simulink model "IEEE34_SPSload"  (R2021b)
settings: Solver=ode4  StartTime=0.0  StopTime=5  FixedStep=50e-6  RelTol=1e-3
PreLoadFcn:
  | pGain = 0.05; % Gain of random perturbation (pu)
  | pGainAP = 0.01; % Gain of sinusoidal active power variation (pu)
  | pGainRP = 0.01; % Gain of sinusoidal reactive power variation (pu)
  | pFreqAP = 0.03; % Frequency of sinusoidal active power variation (Hz)
  | pFreqRP = 0.03; % Frequency of sinusoidal reactive power variation (Hz)
  | 
  | init_IEEE34nodetestfeeder;
InitFcn:
  | pGain = 0.05; % Gain of random perturbation (pu)
  | pGainAP = 0.01; % Gain of sinusoidal active power variation (pu)
  | pGainRP = 0.01; % Gain of sinusoidal reactive power variation (pu)
  | pFreqAP = 0.03; % Frequency of sinusoidal active power variation (Hz)
  | pFreqRP = 0.03; % Frequency of sinusoidal reactive power variation (Hz)
  | 
  | init_IEEE34nodetestfeeder;
values from neighbouring files (symbols this model uses):
  fNom = f    (= 60)    [init_IEEE34nodetestfeeder.m]
  loadcoeff = 1.0    (= 1)    [init_IEEE34nodetestfeeder.m]
  Ts = 50e-6    (= 5e-05)    [init_IEEE34nodetestfeeder.m]
  vNomMV = VsubL    (= 24900)    [init_IEEE34nodetestfeeder.m]
  VsubL = 24.9e3    (= 24900)    [init_IEEE34nodetestfeeder.m]
  VxfmL = 4.16e3    (= 4160)    [init_IEEE34nodetestfeeder.m]
undefined symbols (not defined in the file or in its folder): Ac, Bc, Cc, Dc, find_system, j
libraries: spsSeriesRLCBranchLib x418, spsGroundLib x242, simulink_extras x176, spsVoltageMeasurementLib x106, spsRMSLib x96, spsControlledCurrentSourceLib x94, spsThreePhaseVIMeasurementLib x37, spsMutualInductanceLib x24, spsCurrentMeasurementLib x12, spsOnDelayLib x12, spsLinearTransformerLib x6, spsControlledVoltageSourceLib x6
(part 30 of 33)

== system IEEE34_SPSload/SM_IEEE34/DL_820-822/Load B/model/Positive Sequence current/TF_P ==
  In1 : Inport
  State-Space : StateSpace  A=Ac  B=Bc  C=Cc  D=Dc  InitialCondition=x0c
  Out1 : Outport  VectorParamsAs1DForOutWhenUnconnected=off
  wires:
  State-Space/1 -> Out1/1
  In1/1 -> State-Space/1

== system IEEE34_SPSload/SM_IEEE34/DL_820-822/Load B/model/Positive Sequence current/TF_Q ==
  In1 : Inport
  State-Space : StateSpace  A=Ac  B=Bc  C=Cc  D=Dc  InitialCondition=x0c
  Out1 : Outport  VectorParamsAs1DForOutWhenUnconnected=off
  wires:
  In1/1 -> State-Space/1
  State-Space/1 -> Out1/1

== system IEEE34_SPSload/SM_IEEE34/DL_824-1/Load B/model/PLL/adaptive filter ==
  u : Inport
  freq (Hz) : Inport  Port=2
  Gain : Gain  Gain=2*pi*2*0.707*2
  Gain1 : Gain  Gain=2*pi*2
  Product1 : Product  Inputs=***  RndMeth=Zero
  Product2 : Product  Inputs=**  RndMeth=Zero
  Product3 : Product  Inputs=***  RndMeth=Zero
  Sum1 : Sum  Inputs=+--  InputSameDT=on  SaturateOnIntegerOverflow=on  OutDataTypeStr=Inherit: Same as first input
  integrator1 : Integrator
  integrator2 : Integrator
  y : Outport  VectorParamsAs1DForOutWhenUnconnected=off
  wires:
  Product1/1 -> Sum1/2
  u/1 -> Product3/3
  freq (Hz)/1 -> Gain/1, Gain1/1
  Gain1/1 -> Product1/3, Product1/2, Product3/2, Product3/1
  Product3/1 -> Sum1/1
  integrator1/1 -> Product1/1, y/1
  Gain/1 -> Product2/2
  Product2/1 -> Sum1/3
  Sum1/1 -> integrator2/1
  integrator2/1 -> Product2/1, integrator1/1

== system IEEE34_SPSload/SM_IEEE34/DL_824-1/Load B/model/PLL/adaptive mean ==
  u : Inport
  freq (Hz) : Inport  Port=2
  Fcn : Fcn  Expr=u(1)+1e-6
  Math Function : Math  Operator=reciprocal  SignedPower=on  SaturateOnIntegerOverflow=on
  Product1 : Product  Inputs=**  RndMeth=Zero
  Sum : Sum  Inputs=+-  InputSameDT=on  SaturateOnIntegerOverflow=on  OutDataTypeStr=Inherit: Same as first input
  Variable Transport Delay : VariableTransportDelay  MaximumDelay=1/40  MaximumPoints=4096
  integrator : Integrator
  y : Outport  VectorParamsAs1DForOutWhenUnconnected=off
  wires:
  Product1/1 -> y/1
  u/1 -> integrator/1
  Sum/1 -> Product1/1
  integrator/1 -> Variable Transport Delay/1, Sum/1
  Variable Transport Delay/1 -> Sum/2
  Math Function/1 -> Variable Transport Delay/2
  freq (Hz)/1 -> Fcn/1
  Fcn/1 -> Math Function/1, Product1/2

== system IEEE34_SPSload/SM_IEEE34/DL_824-1/Load B/model/Positive Sequence current/TF_P ==
  In1 : Inport
  State-Space : StateSpace  A=Ac  B=Bc  C=Cc  D=Dc  InitialCondition=x0c
  Out1 : Outport  VectorParamsAs1DForOutWhenUnconnected=off
  wires:
  State-Space/1 -> Out1/1
  In1/1 -> State-Space/1

== system IEEE34_SPSload/SM_IEEE34/DL_824-1/Load B/model/Positive Sequence current/TF_Q ==
  In1 : Inport
  State-Space : StateSpace  A=Ac  B=Bc  C=Cc  D=Dc  InitialCondition=x0c
  Out1 : Outport  VectorParamsAs1DForOutWhenUnconnected=off
  wires:
  In1/1 -> State-Space/1
  State-Space/1 -> Out1/1

== system IEEE34_SPSload/SM_IEEE34/DL_824-2/Load B/model/PLL/adaptive filter ==
  u : Inport
  freq (Hz) : Inport  Port=2
  Gain : Gain  Gain=2*pi*2*0.707*2
  Gain1 : Gain  Gain=2*pi*2
  Product1 : Product  Inputs=***  RndMeth=Zero
  Product2 : Product  Inputs=**  RndMeth=Zero
  Product3 : Product  Inputs=***  RndMeth=Zero
  Sum1 : Sum  Inputs=+--  InputSameDT=on  SaturateOnIntegerOverflow=on  OutDataTypeStr=Inherit: Same as first input
  integrator1 : Integrator
  integrator2 : Integrator
  y : Outport  VectorParamsAs1DForOutWhenUnconnected=off
  wires:
  integrator2/1 -> integrator1/1, Product2/1
  Sum1/1 -> integrator2/1
  Product2/1 -> Sum1/3
  Gain/1 -> Product2/2
  integrator1/1 -> y/1, Product1/1
  Product3/1 -> Sum1/1
  Gain1/1 -> Product3/1, Product3/2, Product1/2, Product1/3
  freq (Hz)/1 -> Gain1/1, Gain/1
  u/1 -> Product3/3
  Product1/1 -> Sum1/2

== system IEEE34_SPSload/SM_IEEE34/DL_824-2/Load B/model/PLL/adaptive mean ==
  u : Inport
  freq (Hz) : Inport  Port=2
  Fcn : Fcn  Expr=u(1)+1e-6
  Math Function : Math  Operator=reciprocal  SignedPower=on  SaturateOnIntegerOverflow=on
  Product1 : Product  Inputs=**  RndMeth=Zero
  Sum : Sum  Inputs=+-  InputSameDT=on  SaturateOnIntegerOverflow=on  OutDataTypeStr=Inherit: Same as first input
  Variable Transport Delay : VariableTransportDelay  MaximumDelay=1/40  MaximumPoints=4096
  integrator : Integrator
  y : Outport  VectorParamsAs1DForOutWhenUnconnected=off
  wires:
  Fcn/1 -> Product1/2, Math Function/1
  freq (Hz)/1 -> Fcn/1
  Math Function/1 -> Variable Transport Delay/2
  Variable Transport Delay/1 -> Sum/2
  integrator/1 -> Sum/1, Variable Transport Delay/1
  Sum/1 -> Product1/1
  u/1 -> integrator/1
  Product1/1 -> y/1

== system IEEE34_SPSload/SM_IEEE34/DL_824-2/Load B/model/Positive Sequence current/TF_P ==
  In1 : Inport
  State-Space : StateSpace  A=Ac  B=Bc  C=Cc  D=Dc  InitialCondition=x0c
  Out1 : Outport  VectorParamsAs1DForOutWhenUnconnected=off
  wires:
  In1/1 -> State-Space/1
  State-Space/1 -> Out1/1

== system IEEE34_SPSload/SM_IEEE34/DL_824-2/Load B/model/Positive Sequence current/TF_Q ==
  In1 : Inport
  State-Space : StateSpace  A=Ac  B=Bc  C=Cc  D=Dc  InitialCondition=x0c
  Out1 : Outport  VectorParamsAs1DForOutWhenUnconnected=off
  wires:
  State-Space/1 -> Out1/1
  In1/1 -> State-Space/1

== system IEEE34_SPSload/SM_IEEE34/DL_824-826/Load B/model/PLL/adaptive filter ==
  u : Inport
  freq (Hz) : Inport  Port=2
  Gain : Gain  Gain=2*pi*2*0.707*2
  Gain1 : Gain  Gain=2*pi*2
  Product1 : Product  Inputs=***  RndMeth=Zero
  Product2 : Product  Inputs=**  RndMeth=Zero
  Product3 : Product  Inputs=***  RndMeth=Zero
  Sum1 : Sum  Inputs=+--  InputSameDT=on  SaturateOnIntegerOverflow=on  OutDataTypeStr=Inherit: Same as first input
  integrator1 : Integrator
  integrator2 : Integrator
  y : Outport  VectorParamsAs1DForOutWhenUnconnected=off
  wires:
  Product1/1 -> Sum1/2
  u/1 -> Product3/3
  freq (Hz)/1 -> Gain/1, Gain1/1
  Gain1/1 -> Product1/3, Product1/2, Product3/2, Product3/1
  Product3/1 -> Sum1/1
  integrator1/1 -> Product1/1, y/1
  Gain/1 -> Product2/2
  Product2/1 -> Sum1/3
  Sum1/1 -> integrator2/1
  integrator2/1 -> Product2/1, integrator1/1

== system IEEE34_SPSload/SM_IEEE34/DL_824-826/Load B/model/PLL/adaptive mean ==
  u : Inport
  freq (Hz) : Inport  Port=2
  Fcn : Fcn  Expr=u(1)+1e-6
  Math Function : Math  Operator=reciprocal  SignedPower=on  SaturateOnIntegerOverflow=on
  Product1 : Product  Inputs=**  RndMeth=Zero
  Sum : Sum  Inputs=+-  InputSameDT=on  SaturateOnIntegerOverflow=on  OutDataTypeStr=Inherit: Same as first input
  Variable Transport Delay : VariableTransportDelay  MaximumDelay=1/40  MaximumPoints=4096
  integrator : Integrator
  y : Outport  VectorParamsAs1DForOutWhenUnconnected=off
  wires:
  Product1/1 -> y/1
  u/1 -> integrator/1
  Sum/1 -> Product1/1
  integrator/1 -> Variable Transport Delay/1, Sum/1
  Variable Transport Delay/1 -> Sum/2
  Math Function/1 -> Variable Transport Delay/2
  freq (Hz)/1 -> Fcn/1
  Fcn/1 -> Math Function/1, Product1/2

== system IEEE34_SPSload/SM_IEEE34/DL_824-826/Load B/model/Positive Sequence current/TF_P ==
  In1 : Inport
  State-Space : StateSpace  A=Ac  B=Bc  C=Cc  D=Dc  InitialCondition=x0c
  Out1 : Outport  VectorParamsAs1DForOutWhenUnconnected=off
  wires:
  State-Space/1 -> Out1/1
  In1/1 -> State-Space/1

== system IEEE34_SPSload/SM_IEEE34/DL_824-826/Load B/model/Positive Sequence current/TF_Q ==
  In1 : Inport
  State-Space : StateSpace  A=Ac  B=Bc  C=Cc  D=Dc  InitialCondition=x0c
  Out1 : Outport  VectorParamsAs1DForOutWhenUnconnected=off
  wires:
  In1/1 -> State-Space/1
  State-Space/1 -> Out1/1

== system IEEE34_SPSload/SM_IEEE34/DL_824-828/Load B/model/PLL/adaptive filter ==
  u : Inport
  freq (Hz) : Inport  Port=2
  Gain : Gain  Gain=2*pi*2*0.707*2
  Gain1 : Gain  Gain=2*pi*2
  Product1 : Product  Inputs=***  RndMeth=Zero
  Product2 : Product  Inputs=**  RndMeth=Zero
  Product3 : Product  Inputs=***  RndMeth=Zero
  Sum1 : Sum  Inputs=+--  InputSameDT=on  SaturateOnIntegerOverflow=on  OutDataTypeStr=Inherit: Same as first input
  integrator1 : Integrator
  integrator2 : Integrator
  y : Outport  VectorParamsAs1DForOutWhenUnconnected=off
  wires:
  Product1/1 -> Sum1/2
  u/1 -> Product3/3
  freq (Hz)/1 -> Gain/1, Gain1/1
  Gain1/1 -> Product1/3, Product1/2, Product3/2, Product3/1
  Product3/1 -> Sum1/1
  integrator1/1 -> Product1/1, y/1
  Gain/1 -> Product2/2
  Product2/1 -> Sum1/3
  Sum1/1 -> integrator2/1
  integrator2/1 -> Product2/1, integrator1/1

== system IEEE34_SPSload/SM_IEEE34/DL_824-828/Load B/model/PLL/adaptive mean ==
  u : Inport
  freq (Hz) : Inport  Port=2
  Fcn : Fcn  Expr=u(1)+1e-6
  Math Function : Math  Operator=reciprocal  SignedPower=on  SaturateOnIntegerOverflow=on
  Product1 : Product  Inputs=**  RndMeth=Zero
  Sum : Sum  Inputs=+-  InputSameDT=on  SaturateOnIntegerOverflow=on  OutDataTypeStr=Inherit: Same as first input
  Variable Transport Delay : VariableTransportDelay  MaximumDelay=1/40  MaximumPoints=4096
  integrator : Integrator
  y : Outport  VectorParamsAs1DForOutWhenUnconnected=off
  wires:
  Product1/1 -> y/1
  u/1 -> integrator/1
  Sum/1 -> Product1/1
  integrator/1 -> Variable Transport Delay/1, Sum/1
  Variable Transport Delay/1 -> Sum/2
  Math Function/1 -> Variable Transport Delay/2
  freq (Hz)/1 -> Fcn/1
  Fcn/1 -> Math Function/1, Product1/2

== system IEEE34_SPSload/SM_IEEE34/DL_824-828/Load B/model/Positive Sequence current/TF_P ==
  In1 : Inport
  State-Space : StateSpace  A=Ac  B=Bc  C=Cc  D=Dc  InitialCondition=x0c
  Out1 : Outport  VectorParamsAs1DForOutWhenUnconnected=off
  wires:
  State-Space/1 -> Out1/1
  In1/1 -> State-Space/1

== system IEEE34_SPSload/SM_IEEE34/DL_824-828/Load B/model/Positive Sequence current/TF_Q ==
  In1 : Inport
  State-Space : StateSpace  A=Ac  B=Bc  C=Cc  D=Dc  InitialCondition=x0c
  Out1 : Outport  VectorParamsAs1DForOutWhenUnconnected=off
  wires:
  In1/1 -> State-Space/1
  State-Space/1 -> Out1/1

== system IEEE34_SPSload/SM_IEEE34/DL_828-1/Load B/model/PLL/adaptive filter ==
  u : Inport
  freq (Hz) : Inport  Port=2
  Gain : Gain  Gain=2*pi*2*0.707*2
  Gain1 : Gain  Gain=2*pi*2
  Product1 : Product  Inputs=***  RndMeth=Zero
  Product2 : Product  Inputs=**  RndMeth=Zero
  Product3 : Product  Inputs=***  RndMeth=Zero
  Sum1 : Sum  Inputs=+--  InputSameDT=on  SaturateOnIntegerOverflow=on  OutDataTypeStr=Inherit: Same as first input
  integrator1 : Integrator
  integrator2 : Integrator
  y : Outport  VectorParamsAs1DForOutWhenUnconnected=off
  wires:
  integrator2/1 -> integrator1/1, Product2/1
  Sum1/1 -> integrator2/1
  Product2/1 -> Sum1/3
  Gain/1 -> Product2/2
  integrator1/1 -> y/1, Product1/1
  Product3/1 -> Sum1/1
  Gain1/1 -> Product3/1, Product3/2, Product1/2, Product1/3
  freq (Hz)/1 -> Gain1/1, Gain/1
  u/1 -> Product3/3
  Product1/1 -> Sum1/2

== system IEEE34_SPSload/SM_IEEE34/DL_828-1/Load B/model/PLL/adaptive mean ==
  u : Inport
  freq (Hz) : Inport  Port=2
  Fcn : Fcn  Expr=u(1)+1e-6
  Math Function : Math  Operator=reciprocal  SignedPower=on  SaturateOnIntegerOverflow=on
  Product1 : Product  Inputs=**  RndMeth=Zero
  Sum : Sum  Inputs=+-  InputSameDT=on  SaturateOnIntegerOverflow=on  OutDataTypeStr=Inherit: Same as first input
  Variable Transport Delay : VariableTransportDelay  MaximumDelay=1/40  MaximumPoints=4096
  integrator : Integrator
  y : Outport  VectorParamsAs1DForOutWhenUnconnected=off
  wires:
  Fcn/1 -> Product1/2, Math Function/1
  freq (Hz)/1 -> Fcn/1
  Math Function/1 -> Variable Transport Delay/2
  Variable Transport Delay/1 -> Sum/2
  integrator/1 -> Sum/1, Variable Transport Delay/1
  Sum/1 -> Product1/1
  u/1 -> integrator/1
  Product1/1 -> y/1

== system IEEE34_SPSload/SM_IEEE34/DL_828-1/Load B/model/Positive Sequence current/TF_P ==
  In1 : Inport
  State-Space : StateSpace  A=Ac  B=Bc  C=Cc  D=Dc  InitialCondition=x0c
  Out1 : Outport  VectorParamsAs1DForOutWhenUnconnected=off
  wires:
  In1/1 -> State-Space/1
  State-Space/1 -> Out1/1

== system IEEE34_SPSload/SM_IEEE34/DL_828-1/Load B/model/Positive Sequence current/TF_Q ==
  In1 : Inport
  State-Space : StateSpace  A=Ac  B=Bc  C=Cc  D=Dc  InitialCondition=x0c
  Out1 : Outport  VectorParamsAs1DForOutWhenUnconnected=off
  wires:
  State-Space/1 -> Out1/1
  In1/1 -> State-Space/1

== system IEEE34_SPSload/SM_IEEE34/DL_828-830/Load B/model/PLL/adaptive filter ==
  u : Inport
  freq (Hz) : Inport  Port=2
  Gain : Gain  Gain=2*pi*2*0.707*2
  Gain1 : Gain  Gain=2*pi*2
  Product1 : Product  Inputs=***  RndMeth=Zero
  Product2 : Product  Inputs=**  RndMeth=Zero
  Product3 : Product  Inputs=***  RndMeth=Zero
  Sum1 : Sum  Inputs=+--  InputSameDT=on  SaturateOnIntegerOverflow=on  OutDataTypeStr=Inherit: Same as first input
  integrator1 : Integrator
  integrator2 : Integrator
  y : Outport  VectorParamsAs1DForOutWhenUnconnected=off
  wires:
  Product1/1 -> Sum1/2
  u/1 -> Product3/3
  freq (Hz)/1 -> Gain/1, Gain1/1
  Gain1/1 -> Product1/3, Product1/2, Product3/2, Product3/1
  Product3/1 -> Sum1/1
  integrator1/1 -> Product1/1, y/1
  Gain/1 -> Product2/2
  Product2/1 -> Sum1/3
  Sum1/1 -> integrator2/1
  integrator2/1 -> Product2/1, integrator1/1

== system IEEE34_SPSload/SM_IEEE34/DL_828-830/Load B/model/PLL/adaptive mean ==
  u : Inport
  freq (Hz) : Inport  Port=2
  Fcn : Fcn  Expr=u(1)+1e-6
  Math Function : Math  Operator=reciprocal  SignedPower=on  SaturateOnIntegerOverflow=on
  Product1 : Product  Inputs=**  RndMeth=Zero
  Sum : Sum  Inputs=+-  InputSameDT=on  SaturateOnIntegerOverflow=on  OutDataTypeStr=Inherit: Same as first input
  Variable Transport Delay : VariableTransportDelay  MaximumDelay=1/40  MaximumPoints=4096
  integrator : Integrator
  y : Outport  VectorParamsAs1DForOutWhenUnconnected=off
  wires:
  Product1/1 -> y/1
  u/1 -> integrator/1
  Sum/1 -> Product1/1
  integrator/1 -> Variable Transport Delay/1, Sum/1
  Variable Transport Delay/1 -> Sum/2
  Math Function/1 -> Variable Transport Delay/2
  freq (Hz)/1 -> Fcn/1
  Fcn/1 -> Math Function/1, Product1/2

== system IEEE34_SPSload/SM_IEEE34/DL_828-830/Load B/model/Positive Sequence current/TF_P ==
  In1 : Inport
  State-Space : StateSpace  A=Ac  B=Bc  C=Cc  D=Dc  InitialCondition=x0c
  Out1 : Outport  VectorParamsAs1DForOutWhenUnconnected=off
  wires:
  State-Space/1 -> Out1/1
  In1/1 -> State-Space/1

== system IEEE34_SPSload/SM_IEEE34/DL_828-830/Load B/model/Positive Sequence current/TF_Q ==
  In1 : Inport
  State-Space : StateSpace  A=Ac  B=Bc  C=Cc  D=Dc  InitialCondition=x0c
  Out1 : Outport  VectorParamsAs1DForOutWhenUnconnected=off
  wires:
  In1/1 -> State-Space/1
  State-Space/1 -> Out1/1

== system IEEE34_SPSload/SM_IEEE34/DL_832-1/Load A/model/PLL/adaptive filter ==
  u : Inport
  freq (Hz) : Inport  Port=2
  Gain : Gain  Gain=2*pi*2*0.707*2
  Gain1 : Gain  Gain=2*pi*2
  Product1 : Product  Inputs=***  RndMeth=Zero
  Product2 : Product  Inputs=**  RndMeth=Zero
  Product3 : Product  Inputs=***  RndMeth=Zero
  Sum1 : Sum  Inputs=+--  InputSameDT=on  SaturateOnIntegerOverflow=on  OutDataTypeStr=Inherit: Same as first input
  integrator1 : Integrator
  integrator2 : Integrator
  y : Outport  VectorParamsAs1DForOutWhenUnconnected=off
  wires:
  integrator2/1 -> integrator1/1, Product2/1
  Sum1/1 -> integrator2/1
  Product2/1 -> Sum1/3
  Gain/1 -> Product2/2
  integrator1/1 -> y/1, Product1/1
  Product3/1 -> Sum1/1
  Gain1/1 -> Product3/1, Product3/2, Product1/2, Product1/3
  freq (Hz)/1 -> Gain1/1, Gain/1
  u/1 -> Product3/3
  Product1/1 -> Sum1/2

== system IEEE34_SPSload/SM_IEEE34/DL_832-1/Load A/model/PLL/adaptive mean ==
  u : Inport
  freq (Hz) : Inport  Port=2
  Fcn : Fcn  Expr=u(1)+1e-6
  Math Function : Math  Operator=reciprocal  SignedPower=on  SaturateOnIntegerOverflow=on
  Product1 : Product  Inputs=**  RndMeth=Zero
  Sum : Sum  Inputs=+-  InputSameDT=on  SaturateOnIntegerOverflow=on  OutDataTypeStr=Inherit: Same as first input
  Variable Transport Delay : VariableTransportDelay  MaximumDelay=1/40  MaximumPoints=4096
  integrator : Integrator
  y : Outport  VectorParamsAs1DForOutWhenUnconnected=off
  wires:
  Fcn/1 -> Product1/2, Math Function/1
  freq (Hz)/1 -> Fcn/1
  Math Function/1 -> Variable Transport Delay/2
  Variable Transport Delay/1 -> Sum/2
  integrator/1 -> Sum/1, Variable Transport Delay/1
  Sum/1 -> Product1/1
  u/1 -> integrator/1
  Product1/1 -> y/1

== system IEEE34_SPSload/SM_IEEE34/DL_832-1/Load A/model/Positive Sequence current/TF_P ==
  In1 : Inport
  State-Space : StateSpace  A=Ac  B=Bc  C=Cc  D=Dc  InitialCondition=x0c
  Out1 : Outport  VectorParamsAs1DForOutWhenUnconnected=off
  wires:
  In1/1 -> State-Space/1
  State-Space/1 -> Out1/1

== system IEEE34_SPSload/SM_IEEE34/DL_832-1/Load A/model/Positive Sequence current/TF_Q ==
  In1 : Inport
  State-Space : StateSpace  A=Ac  B=Bc  C=Cc  D=Dc  InitialCondition=x0c
  Out1 : Outport  VectorParamsAs1DForOutWhenUnconnected=off
  wires:
  State-Space/1 -> Out1/1
  In1/1 -> State-Space/1

== system IEEE34_SPSload/SM_IEEE34/DL_832-1/Load B/model/PLL/adaptive filter ==
  u : Inport
  freq (Hz) : Inport  Port=2
  Gain : Gain  Gain=2*pi*2*0.707*2
  Gain1 : Gain  Gain=2*pi*2
  Product1 : Product  Inputs=***  RndMeth=Zero
  Product2 : Product  Inputs=**  RndMeth=Zero
  Product3 : Product  Inputs=***  RndMeth=Zero
  Sum1 : Sum  Inputs=+--  InputSameDT=on  SaturateOnIntegerOverflow=on  OutDataTypeStr=Inherit: Same as first input
  integrator1 : Integrator
  integrator2 : Integrator
  y : Outport  VectorParamsAs1DForOutWhenUnconnected=off
  wires:
  Product1/1 -> Sum1/2
  u/1 -> Product3/3
  freq (Hz)/1 -> Gain/1, Gain1/1
  Gain1/1 -> Product1/3, Product1/2, Product3/2, Product3/1
  Product3/1 -> Sum1/1
  integrator1/1 -> Product1/1, y/1
  Gain/1 -> Product2/2
  Product2/1 -> Sum1/3
  Sum1/1 -> integrator2/1
  integrator2/1 -> Product2/1, integrator1/1

== system IEEE34_SPSload/SM_IEEE34/DL_832-1/Load B/model/PLL/adaptive mean ==
  u : Inport
  freq (Hz) : Inport  Port=2
  Fcn : Fcn  Expr=u(1)+1e-6
  Math Function : Math  Operator=reciprocal  SignedPower=on  SaturateOnIntegerOverflow=on
  Product1 : Product  Inputs=**  RndMeth=Zero
  Sum : Sum  Inputs=+-  InputSameDT=on  SaturateOnIntegerOverflow=on  OutDataTypeStr=Inherit: Same as first input
  Variable Transport Delay : VariableTransportDelay  MaximumDelay=1/40  MaximumPoints=4096
  integrator : Integrator
  y : Outport  VectorParamsAs1DForOutWhenUnconnected=off
  wires:
  Product1/1 -> y/1
  u/1 -> integrator/1
  Sum/1 -> Product1/1
  integrator/1 -> Variable Transport Delay/1, Sum/1
  Variable Transport Delay/1 -> Sum/2
  Math Function/1 -> Variable Transport Delay/2
  freq (Hz)/1 -> Fcn/1
  Fcn/1 -> Math Function/1, Product1/2

== system IEEE34_SPSload/SM_IEEE34/DL_832-1/Load B/model/Positive Sequence current/TF_P ==
  In1 : Inport
  State-Space : StateSpace  A=Ac  B=Bc  C=Cc  D=Dc  InitialCondition=x0c
  Out1 : Outport  VectorParamsAs1DForOutWhenUnconnected=off
  wires:
  State-Space/1 -> Out1/1
  In1/1 -> State-Space/1

== system IEEE34_SPSload/SM_IEEE34/DL_832-1/Load B/model/Positive Sequence current/TF_Q ==
  In1 : Inport
  State-Space : StateSpace  A=Ac  B=Bc  C=Cc  D=Dc  InitialCondition=x0c
  Out1 : Outport  VectorParamsAs1DForOutWhenUnconnected=off
  wires:
  In1/1 -> State-Space/1
  State-Space/1 -> Out1/1

== system IEEE34_SPSload/SM_IEEE34/DL_832-1/Load C/model/PLL/adaptive filter ==
  u : Inport
  freq (Hz) : Inport  Port=2
  Gain : Gain  Gain=2*pi*2*0.707*2
  Gain1 : Gain  Gain=2*pi*2
  Product1 : Product  Inputs=***  RndMeth=Zero
  Product2 : Product  Inputs=**  RndMeth=Zero
  Product3 : Product  Inputs=***  RndMeth=Zero
  Sum1 : Sum  Inputs=+--  InputSameDT=on  SaturateOnIntegerOverflow=on  OutDataTypeStr=Inherit: Same as first input
  integrator1 : Integrator
  integrator2 : Integrator
  y : Outport  VectorParamsAs1DForOutWhenUnconnected=off
  wires:
  integrator2/1 -> integrator1/1, Product2/1
  Sum1/1 -> integrator2/1
  Product2/1 -> Sum1/3
  Gain/1 -> Product2/2
  integrator1/1 -> y/1, Product1/1
  Product3/1 -> Sum1/1
  Gain1/1 -> Product3/1, Product3/2, Product1/2, Product1/3
  freq (Hz)/1 -> Gain1/1, Gain/1
  u/1 -> Product3/3
  Product1/1 -> Sum1/2

== system IEEE34_SPSload/SM_IEEE34/DL_832-1/Load C/model/PLL/adaptive mean ==
  u : Inport
  freq (Hz) : Inport  Port=2
  Fcn : Fcn  Expr=u(1)+1e-6
  Math Function : Math  Operator=reciprocal  SignedPower=on  SaturateOnIntegerOverflow=on
  Product1 : Product  Inputs=**  RndMeth=Zero
  Sum : Sum  Inputs=+-  InputSameDT=on  SaturateOnIntegerOverflow=on  OutDataTypeStr=Inherit: Same as first input
  Variable Transport Delay : VariableTransportDelay  MaximumDelay=1/40  MaximumPoints=4096
  integrator : Integrator
  y : Outport  VectorParamsAs1DForOutWhenUnconnected=off
  wires:
  Fcn/1 -> Product1/2, Math Function/1
  freq (Hz)/1 -> Fcn/1
  Math Function/1 -> Variable Transport Delay/2
  Variable Transport Delay/1 -> Sum/2
  integrator/1 -> Sum/1, Variable Transport Delay/1
  Sum/1 -> Product1/1
  u/1 -> integrator/1
  Product1/1 -> y/1

== system IEEE34_SPSload/SM_IEEE34/DL_832-1/Load C/model/Positive Sequence current/TF_P ==
  In1 : Inport
  State-Space : StateSpace  A=Ac  B=Bc  C=Cc  D=Dc  InitialCondition=x0c
  Out1 : Outport  VectorParamsAs1DForOutWhenUnconnected=off
  wires:
  In1/1 -> State-Space/1
  State-Space/1 -> Out1/1

== system IEEE34_SPSload/SM_IEEE34/DL_832-1/Load C/model/Positive Sequence current/TF_Q ==
  In1 : Inport
  State-Space : StateSpace  A=Ac  B=Bc  C=Cc  D=Dc  InitialCondition=x0c
  Out1 : Outport  VectorParamsAs1DForOutWhenUnconnected=off
  wires:
  State-Space/1 -> Out1/1
  In1/1 -> State-Space/1

== system IEEE34_SPSload/SM_IEEE34/DL_832-858/Load A/model/PLL/adaptive filter ==
  u : Inport
  freq (Hz) : Inport  Port=2
  Gain : Gain  Gain=2*pi*2*0.707*2
  Gain1 : Gain  Gain=2*pi*2
  Product1 : Product  Inputs=***  RndMeth=Zero
  Product2 : Product  Inputs=**  RndMeth=Zero
  Product3 : Product  Inputs=***  RndMeth=Zero
  Sum1 : Sum  Inputs=+--  InputSameDT=on  SaturateOnIntegerOverflow=on  OutDataTypeStr=Inherit: Same as first input
  integrator1 : Integrator
  integrator2 : Integrator
  y : Outport  VectorParamsAs1DForOutWhenUnconnected=off
  wires:
  Product1/1 -> Sum1/2
  u/1 -> Product3/3
  freq (Hz)/1 -> Gain/1, Gain1/1
  Gain1/1 -> Product1/3, Product1/2, Product3/2, Product3/1
  Product3/1 -> Sum1/1
  integrator1/1 -> Product1/1, y/1
  Gain/1 -> Product2/2
  Product2/1 -> Sum1/3
  Sum1/1 -> integrator2/1
  integrator2/1 -> Product2/1, integrator1/1

== system IEEE34_SPSload/SM_IEEE34/DL_832-858/Load A/model/PLL/adaptive mean ==
  u : Inport
  freq (Hz) : Inport  Port=2
  Fcn : Fcn  Expr=u(1)+1e-6
  Math Function : Math  Operator=reciprocal  SignedPower=on  SaturateOnIntegerOverflow=on
  Product1 : Product  Inputs=**  RndMeth=Zero
  Sum : Sum  Inputs=+-  InputSameDT=on  SaturateOnIntegerOverflow=on  OutDataTypeStr=Inherit: Same as first input
  Variable Transport Delay : VariableTransportDelay  MaximumDelay=1/40  MaximumPoints=4096
  integrator : Integrator
  y : Outport  VectorParamsAs1DForOutWhenUnconnected=off
  wires:
  Product1/1 -> y/1
  u/1 -> integrator/1
  Sum/1 -> Product1/1
  integrator/1 -> Variable Transport Delay/1, Sum/1
  Variable Transport Delay/1 -> Sum/2
  Math Function/1 -> Variable Transport Delay/2
  freq (Hz)/1 -> Fcn/1
  Fcn/1 -> Math Function/1, Product1/2

== system IEEE34_SPSload/SM_IEEE34/DL_832-858/Load A/model/Positive Sequence current/TF_P ==
  In1 : Inport
  State-Space : StateSpace  A=Ac  B=Bc  C=Cc  D=Dc  InitialCondition=x0c
  Out1 : Outport  VectorParamsAs1DForOutWhenUnconnected=off
  wires:
  State-Space/1 -> Out1/1
  In1/1 -> State-Space/1

== system IEEE34_SPSload/SM_IEEE34/DL_832-858/Load A/model/Positive Sequence current/TF_Q ==
  In1 : Inport
  State-Space : StateSpace  A=Ac  B=Bc  C=Cc  D=Dc  InitialCondition=x0c
  Out1 : Outport  VectorParamsAs1DForOutWhenUnconnected=off
  wires:
  In1/1 -> State-Space/1
  State-Space/1 -> Out1/1

== system IEEE34_SPSload/SM_IEEE34/DL_832-858/Load B/model/PLL/adaptive filter ==
  u : Inport
  freq (Hz) : Inport  Port=2
  Gain : Gain  Gain=2*pi*2*0.707*2
  Gain1 : Gain  Gain=2*pi*2
  Product1 : Product  Inputs=***  RndMeth=Zero
  Product2 : Product  Inputs=**  RndMeth=Zero
  Product3 : Product  Inputs=***  RndMeth=Zero
  Sum1 : Sum  Inputs=+--  InputSameDT=on  SaturateOnIntegerOverflow=on  OutDataTypeStr=Inherit: Same as first input
  integrator1 : Integrator
  integrator2 : Integrator
  y : Outport  VectorParamsAs1DForOutWhenUnconnected=off
  wires:
  integrator2/1 -> integrator1/1, Product2/1
  Sum1/1 -> integrator2/1
  Product2/1 -> Sum1/3
  Gain/1 -> Product2/2
  integrator1/1 -> y/1, Product1/1
  Product3/1 -> Sum1/1
  Gain1/1 -> Product3/1, Product3/2, Product1/2, Product1/3
  freq (Hz)/1 -> Gain1/1, Gain/1
  u/1 -> Product3/3
  Product1/1 -> Sum1/2

== system IEEE34_SPSload/SM_IEEE34/DL_832-858/Load B/model/PLL/adaptive mean ==
  u : Inport
  freq (Hz) : Inport  Port=2
  Fcn : Fcn  Expr=u(1)+1e-6
  Math Function : Math  Operator=reciprocal  SignedPower=on  SaturateOnIntegerOverflow=on
  Product1 : Product  Inputs=**  RndMeth=Zero
  Sum : Sum  Inputs=+-  InputSameDT=on  SaturateOnIntegerOverflow=on  OutDataTypeStr=Inherit: Same as first input
  Variable Transport Delay : VariableTransportDelay  MaximumDelay=1/40  MaximumPoints=4096
  integrator : Integrator
  y : Outport  VectorParamsAs1DForOutWhenUnconnected=off
  wires:
  Fcn/1 -> Product1/2, Math Function/1
  freq (Hz)/1 -> Fcn/1
  Math Function/1 -> Variable Transport Delay/2
  Variable Transport Delay/1 -> Sum/2
  integrator/1 -> Sum/1, Variable Transport Delay/1
  Sum/1 -> Product1/1
  u/1 -> integrator/1
  Product1/1 -> y/1

== system IEEE34_SPSload/SM_IEEE34/DL_832-858/Load B/model/Positive Sequence current/TF_P ==
  In1 : Inport
  State-Space : StateSpace  A=Ac  B=Bc  C=Cc  D=Dc  InitialCondition=x0c
  Out1 : Outport  VectorParamsAs1DForOutWhenUnconnected=off
  wires:
  In1/1 -> State-Space/1
  State-Space/1 -> Out1/1

== system IEEE34_SPSload/SM_IEEE34/DL_832-858/Load B/model/Positive Sequence current/TF_Q ==
  In1 : Inport
  State-Space : StateSpace  A=Ac  B=Bc  C=Cc  D=Dc  InitialCondition=x0c
  Out1 : Outport  VectorParamsAs1DForOutWhenUnconnected=off
  wires:
  State-Space/1 -> Out1/1
  In1/1 -> State-Space/1

== system IEEE34_SPSload/SM_IEEE34/DL_832-858/Load C/model/PLL/adaptive filter ==
  u : Inport
  freq (Hz) : Inport  Port=2
  Gain : Gain  Gain=2*pi*2*0.707*2
  Gain1 : Gain  Gain=2*pi*2
  Product1 : Product  Inputs=***  RndMeth=Zero
  Product2 : Product  Inputs=**  RndMeth=Zero
  Product3 : Product  Inputs=***  RndMeth=Zero
  Sum1 : Sum  Inputs=+--  InputSameDT=on  SaturateOnIntegerOverflow=on  OutDataTypeStr=Inherit: Same as first input
  integrator1 : Integrator
  integrator2 : Integrator
  y : Outport  VectorParamsAs1DForOutWhenUnconnected=off
  wires:
  Product1/1 -> Sum1/2
  u/1 -> Product3/3
  freq (Hz)/1 -> Gain/1, Gain1/1
  Gain1/1 -> Product1/3, Product1/2, Product3/2, Product3/1
  Product3/1 -> Sum1/1
  integrator1/1 -> Product1/1, y/1
  Gain/1 -> Product2/2
  Product2/1 -> Sum1/3
  Sum1/1 -> integrator2/1
  integrator2/1 -> Product2/1, integrator1/1

== system IEEE34_SPSload/SM_IEEE34/DL_832-858/Load C/model/PLL/adaptive mean ==
  u : Inport
  freq (Hz) : Inport  Port=2
  Fcn : Fcn  Expr=u(1)+1e-6
  Math Function : Math  Operator=reciprocal  SignedPower=on  SaturateOnIntegerOverflow=on
  Product1 : Product  Inputs=**  RndMeth=Zero
  Sum : Sum  Inputs=+-  InputSameDT=on  SaturateOnIntegerOverflow=on  OutDataTypeStr=Inherit: Same as first input
  Variable Transport Delay : VariableTransportDelay  MaximumDelay=1/40  MaximumPoints=4096
  integrator : Integrator
  y : Outport  VectorParamsAs1DForOutWhenUnconnected=off
  wires:
  Product1/1 -> y/1
  u/1 -> integrator/1
  Sum/1 -> Product1/1
  integrator/1 -> Variable Transport Delay/1, Sum/1
  Variable Transport Delay/1 -> Sum/2
  Math Function/1 -> Variable Transport Delay/2
  freq (Hz)/1 -> Fcn/1
  Fcn/1 -> Math Function/1, Product1/2

== system IEEE34_SPSload/SM_IEEE34/DL_832-858/Load C/model/Positive Sequence current/TF_P ==
  In1 : Inport
  State-Space : StateSpace  A=Ac  B=Bc  C=Cc  D=Dc  InitialCondition=x0c
  Out1 : Outport  VectorParamsAs1DForOutWhenUnconnected=off
  wires:
  State-Space/1 -> Out1/1
  In1/1 -> State-Space/1

== system IEEE34_SPSload/SM_IEEE34/DL_832-858/Load C/model/Positive Sequence current/TF_Q ==
  In1 : Inport
  State-Space : StateSpace  A=Ac  B=Bc  C=Cc  D=Dc  InitialCondition=x0c
  Out1 : Outport  VectorParamsAs1DForOutWhenUnconnected=off
  wires:
  In1/1 -> State-Space/1
  State-Space/1 -> Out1/1

== system IEEE34_SPSload/SM_IEEE34/DL_834-1/Load B/model/PLL/adaptive filter ==
  u : Inport
  freq (Hz) : Inport  Port=2
  Gain : Gain  Gain=2*pi*2*0.707*2
  Gain1 : Gain  Gain=2*pi*2
  Product1 : Product  Inputs=***  RndMeth=Zero
  Product2 : Product  Inputs=**  RndMeth=Zero
  Product3 : Product  Inputs=***  RndMeth=Zero
  Sum1 : Sum  Inputs=+--  InputSameDT=on  SaturateOnIntegerOverflow=on  OutDataTypeStr=Inherit: Same as first input
  integrator1 : Integrator
  integrator2 : Integrator
  y : Outport  VectorParamsAs1DForOutWhenUnconnected=off
  wires:
  integrator2/1 -> integrator1/1, Product2/1
  Sum1/1 -> integrator2/1
  Product2/1 -> Sum1/3
  Gain/1 -> Product2/2
  integrator1/1 -> y/1, Product1/1
  Product3/1 -> Sum1/1
  Gain1/1 -> Product3/1, Product3/2, Product1/2, Product1/3
  freq (Hz)/1 -> Gain1/1, Gain/1
  u/1 -> Product3/3
  Product1/1 -> Sum1/2

== system IEEE34_SPSload/SM_IEEE34/DL_834-1/Load B/model/PLL/adaptive mean ==
  u : Inport
  freq (Hz) : Inport  Port=2
  Fcn : Fcn  Expr=u(1)+1e-6
  Math Function : Math  Operator=reciprocal  SignedPower=on  SaturateOnIntegerOverflow=on
  Product1 : Product  Inputs=**  RndMeth=Zero
  Sum : Sum  Inputs=+-  InputSameDT=on  SaturateOnIntegerOverflow=on  OutDataTypeStr=Inherit: Same as first input
  Variable Transport Delay : VariableTransportDelay  MaximumDelay=1/40  MaximumPoints=4096
  integrator : Integrator
  y : Outport  VectorParamsAs1DForOutWhenUnconnected=off
  wires:
  Fcn/1 -> Product1/2, Math Function/1
  freq (Hz)/1 -> Fcn/1
  Math Function/1 -> Variable Transport Delay/2
  Variable Transport Delay/1 -> Sum/2
  integrator/1 -> Sum/1, Variable Transport Delay/1
  Sum/1 -> Product1/1
  u/1 -> integrator/1
  Product1/1 -> y/1

== system IEEE34_SPSload/SM_IEEE34/DL_834-1/Load B/model/Positive Sequence current/TF_P ==
  In1 : Inport
  State-Space : StateSpace  A=Ac  B=Bc  C=Cc  D=Dc  InitialCondition=x0c
  Out1 : Outport  VectorParamsAs1DForOutWhenUnconnected=off
  wires:
  In1/1 -> State-Space/1
  State-Space/1 -> Out1/1

== system IEEE34_SPSload/SM_IEEE34/DL_834-1/Load B/model/Positive Sequence current/TF_Q ==
  In1 : Inport
  State-Space : StateSpace  A=Ac  B=Bc  C=Cc  D=Dc  InitialCondition=x0c
  Out1 : Outport  VectorParamsAs1DForOutWhenUnconnected=off
  wires:
  State-Space/1 -> Out1/1
  In1/1 -> State-Space/1

== system IEEE34_SPSload/SM_IEEE34/DL_834-1/Load B1/model/PLL/adaptive filter ==
  u : Inport
  freq (Hz) : Inport  Port=2
  Gain : Gain  Gain=2*pi*2*0.707*2
  Gain1 : Gain  Gain=2*pi*2
  Product1 : Product  Inputs=***  RndMeth=Zero
  Product2 : Product  Inputs=**  RndMeth=Zero
  Product3 : Product  Inputs=***  RndMeth=Zero
  Sum1 : Sum  Inputs=+--  InputSameDT=on  SaturateOnIntegerOverflow=on  OutDataTypeStr=Inherit: Same as first input
  integrator1 : Integrator
  integrator2 : Integrator
  y : Outport  VectorParamsAs1DForOutWhenUnconnected=off
  wires:
  integrator2/1 -> integrator1/1, Product2/1
  Sum1/1 -> integrator2/1
  Product2/1 -> Sum1/3
  Gain/1 -> Product2/2
  integrator1/1 -> y/1, Product1/1
  Product3/1 -> Sum1/1
  Gain1/1 -> Product3/1, Product3/2, Product1/2, Product1/3
  freq (Hz)/1 -> Gain1/1, Gain/1
  u/1 -> Product3/3
  Product1/1 -> Sum1/2

== system IEEE34_SPSload/SM_IEEE34/DL_834-1/Load B1/model/PLL/adaptive mean ==
  u : Inport
  freq (Hz) : Inport  Port=2
  Fcn : Fcn  Expr=u(1)+1e-6
  Math Function : Math  Operator=reciprocal  SignedPower=on  SaturateOnIntegerOverflow=on
  Product1 : Product  Inputs=**  RndMeth=Zero
  Sum : Sum  Inputs=+-  InputSameDT=on  SaturateOnIntegerOverflow=on  OutDataTypeStr=Inherit: Same as first input
  Variable Transport Delay : VariableTransportDelay  MaximumDelay=1/40  MaximumPoints=4096
  integrator : Integrator
  y : Outport  VectorParamsAs1DForOutWhenUnconnected=off
  wires:
  Fcn/1 -> Product1/2, Math Function/1
  freq (Hz)/1 -> Fcn/1
  Math Function/1 -> Variable Transport Delay/2
  Variable Transport Delay/1 -> Sum/2
  integrator/1 -> Sum/1, Variable Transport Delay/1
  Sum/1 -> Product1/1
  u/1 -> integrator/1
  Product1/1 -> y/1

== system IEEE34_SPSload/SM_IEEE34/DL_834-1/Load B1/model/Positive Sequence current/TF_P ==
  In1 : Inport
  State-Space : StateSpace  A=Ac  B=Bc  C=Cc  D=Dc  InitialCondition=x0c
  Out1 : Outport  VectorParamsAs1DForOutWhenUnconnected=off
  wires:
  In1/1 -> State-Space/1
  State-Space/1 -> Out1/1

== system IEEE34_SPSload/SM_IEEE34/DL_834-1/Load B1/model/Positive Sequence current/TF_Q ==
  In1 : Inport
  State-Space : StateSpace  A=Ac  B=Bc  C=Cc  D=Dc  InitialCondition=x0c
  Out1 : Outport  VectorParamsAs1DForOutWhenUnconnected=off
  wires:
  State-Space/1 -> Out1/1
  In1/1 -> State-Space/1

== system IEEE34_SPSload/SM_IEEE34/DL_834-1/Load B2/model/PLL/adaptive filter ==
  u : Inport
  freq (Hz) : Inport  Port=2
  Gain : Gain  Gain=2*pi*2*0.707*2
  Gain1 : Gain  Gain=2*pi*2
  Product1 : Product  Inputs=***  RndMeth=Zero
  Product2 : Product  Inputs=**  RndMeth=Zero
  Product3 : Product  Inputs=***  RndMeth=Zero
  Sum1 : Sum  Inputs=+--  InputSameDT=on  SaturateOnIntegerOverflow=on  OutDataTypeStr=Inherit: Same as first input
  integrator1 : Integrator
  integrator2 : Integrator
  y : Outport  VectorParamsAs1DForOutWhenUnconnected=off
  wires:
  integrator2/1 -> integrator1/1, Product2/1
  Sum1/1 -> integrator2/1
  Product2/1 -> Sum1/3
  Gain/1 -> Product2/2
  integrator1/1 -> y/1, Product1/1
  Product3/1 -> Sum1/1
  Gain1/1 -> Product3/1, Product3/2, Product1/2, Product1/3
  freq (Hz)/1 -> Gain1/1, Gain/1
  u/1 -> Product3/3
  Product1/1 -> Sum1/2

== system IEEE34_SPSload/SM_IEEE34/DL_834-1/Load B2/model/PLL/adaptive mean ==
  u : Inport
  freq (Hz) : Inport  Port=2
  Fcn : Fcn  Expr=u(1)+1e-6
  Math Function : Math  Operator=reciprocal  SignedPower=on  SaturateOnIntegerOverflow=on
  Product1 : Product  Inputs=**  RndMeth=Zero
  Sum : Sum  Inputs=+-  InputSameDT=on  SaturateOnIntegerOverflow=on  OutDataTypeStr=Inherit: Same as first input
  Variable Transport Delay : VariableTransportDelay  MaximumDelay=1/40  MaximumPoints=4096
  integrator : Integrator
  y : Outport  VectorParamsAs1DForOutWhenUnconnected=off
  wires:
  Fcn/1 -> Product1/2, Math Function/1
  freq (Hz)/1 -> Fcn/1
  Math Function/1 -> Variable Transport Delay/2
  Variable Transport Delay/1 -> Sum/2
  integrator/1 -> Sum/1, Variable Transport Delay/1
  Sum/1 -> Product1/1
  u/1 -> integrator/1
  Product1/1 -> y/1

== system IEEE34_SPSload/SM_IEEE34/DL_834-1/Load B2/model/Positive Sequence current/TF_P ==
  In1 : Inport
  State-Space : StateSpace  A=Ac  B=Bc  C=Cc  D=Dc  InitialCondition=x0c
  Out1 : Outport  VectorParamsAs1DForOutWhenUnconnected=off
  wires:
  In1/1 -> State-Space/1
  State-Space/1 -> Out1/1

== system IEEE34_SPSload/SM_IEEE34/DL_834-1/Load B2/model/Positive Sequence current/TF_Q ==
  In1 : Inport
  State-Space : StateSpace  A=Ac  B=Bc  C=Cc  D=Dc  InitialCondition=x0c
  Out1 : Outport  VectorParamsAs1DForOutWhenUnconnected=off
  wires:
  State-Space/1 -> Out1/1
  In1/1 -> State-Space/1

== system IEEE34_SPSload/SM_IEEE34/DL_834-860/Load B/model/PLL/adaptive filter ==
  u : Inport
  freq (Hz) : Inport  Port=2
  Gain : Gain  Gain=2*pi*2*0.707*2
  Gain1 : Gain  Gain=2*pi*2
  Product1 : Product  Inputs=***  RndMeth=Zero
  Product2 : Product  Inputs=**  RndMeth=Zero
  Product3 : Product  Inputs=***  RndMeth=Zero
  Sum1 : Sum  Inputs=+--  InputSameDT=on  SaturateOnIntegerOverflow=on  OutDataTypeStr=Inherit: Same as first input
  integrator1 : Integrator
  integrator2 : Integrator
  y : Outport  VectorParamsAs1DForOutWhenUnconnected=off
  wires:
  Product1/1 -> Sum1/2
  u/1 -> Product3/3
  freq (Hz)/1 -> Gain/1, Gain1/1
  Gain1/1 -> Product1/3, Product1/2, Product3/2, Product3/1
  Product3/1 -> Sum1/1
  integrator1/1 -> Product1/1, y/1
  Gain/1 -> Product2/2
  Product2/1 -> Sum1/3
  Sum1/1 -> integrator2/1
  integrator2/1 -> Product2/1, integrator1/1

== system IEEE34_SPSload/SM_IEEE34/DL_834-860/Load B/model/PLL/adaptive mean ==
  u : Inport
  freq (Hz) : Inport  Port=2
  Fcn : Fcn  Expr=u(1)+1e-6
  Math Function : Math  Operator=reciprocal  SignedPower=on  SaturateOnIntegerOverflow=on
  Product1 : Product  Inputs=**  RndMeth=Zero
  Sum : Sum  Inputs=+-  InputSameDT=on  SaturateOnIntegerOverflow=on  OutDataTypeStr=Inherit: Same as first input
  Variable Transport Delay : VariableTransportDelay  MaximumDelay=1/40  MaximumPoints=4096
  integrator : Integrator
  y : Outport  VectorParamsAs1DForOutWhenUnconnected=off
  wires:
  Product1/1 -> y/1
  u/1 -> integrator/1
  Sum/1 -> Product1/1
  integrator/1 -> Variable Transport Delay/1, Sum/1
  Variable Transport Delay/1 -> Sum/2
  Math Function/1 -> Variable Transport Delay/2
  freq (Hz)/1 -> Fcn/1
  Fcn/1 -> Math Function/1, Product1/2

== system IEEE34_SPSload/SM_IEEE34/DL_834-860/Load B/model/Positive Sequence current/TF_P ==
  In1 : Inport
  State-Space : StateSpace  A=Ac  B=Bc  C=Cc  D=Dc  InitialCondition=x0c
  Out1 : Outport  VectorParamsAs1DForOutWhenUnconnected=off
  wires:
  State-Space/1 -> Out1/1
  In1/1 -> State-Space/1

== system IEEE34_SPSload/SM_IEEE34/DL_834-860/Load B/model/Positive Sequence current/TF_Q ==
  In1 : Inport
  State-Space : StateSpace  A=Ac  B=Bc  C=Cc  D=Dc  InitialCondition=x0c
  Out1 : Outport  VectorParamsAs1DForOutWhenUnconnected=off
  wires:
  In1/1 -> State-Space/1
  State-Space/1 -> Out1/1

== system IEEE34_SPSload/SM_IEEE34/DL_834-860/Load B1/model/PLL/adaptive filter ==
  u : Inport
  freq (Hz) : Inport  Port=2
  Gain : Gain  Gain=2*pi*2*0.707*2
  Gain1 : Gain  Gain=2*pi*2
  Product1 : Product  Inputs=***  RndMeth=Zero
  Product2 : Product  Inputs=**  RndMeth=Zero
  Product3 : Product  Inputs=***  RndMeth=Zero
  Sum1 : Sum  Inputs=+--  InputSameDT=on  SaturateOnIntegerOverflow=on  OutDataTypeStr=Inherit: Same as first input
  integrator1 : Integrator
  integrator2 : Integrator
  y : Outport  VectorParamsAs1DForOutWhenUnconnected=off
  wires:
  Product1/1 -> Sum1/2
  u/1 -> Product3/3
  freq (Hz)/1 -> Gain/1, Gain1/1
  Gain1/1 -> Product1/3, Product1/2, Product3/2, Product3/1
  Product3/1 -> Sum1/1
  integrator1/1 -> Product1/1, y/1
  Gain/1 -> Product2/2
  Product2/1 -> Sum1/3
  Sum1/1 -> integrator2/1
  integrator2/1 -> Product2/1, integrator1/1

== system IEEE34_SPSload/SM_IEEE34/DL_834-860/Load B1/model/PLL/adaptive mean ==
  u : Inport
  freq (Hz) : Inport  Port=2
  Fcn : Fcn  Expr=u(1)+1e-6
  Math Function : Math  Operator=reciprocal  SignedPower=on  SaturateOnIntegerOverflow=on
  Product1 : Product  Inputs=**  RndMeth=Zero
  Sum : Sum  Inputs=+-  InputSameDT=on  SaturateOnIntegerOverflow=on  OutDataTypeStr=Inherit: Same as first input
  Variable Transport Delay : VariableTransportDelay  MaximumDelay=1/40  MaximumPoints=4096
  integrator : Integrator
  y : Outport  VectorParamsAs1DForOutWhenUnconnected=off
  wires:
  Product1/1 -> y/1
  u/1 -> integrator/1
  Sum/1 -> Product1/1
  integrator/1 -> Variable Transport Delay/1, Sum/1
  Variable Transport Delay/1 -> Sum/2
  Math Function/1 -> Variable Transport Delay/2
  freq (Hz)/1 -> Fcn/1
  Fcn/1 -> Math Function/1, Product1/2

== system IEEE34_SPSload/SM_IEEE34/DL_834-860/Load B1/model/Positive Sequence current/TF_P ==
  In1 : Inport
  State-Space : StateSpace  A=Ac  B=Bc  C=Cc  D=Dc  InitialCondition=x0c
  Out1 : Outport  VectorParamsAs1DForOutWhenUnconnected=off
  wires:
  State-Space/1 -> Out1/1
  In1/1 -> State-Space/1

== system IEEE34_SPSload/SM_IEEE34/DL_834-860/Load B1/model/Positive Sequence current/TF_Q ==
  In1 : Inport
  State-Space : StateSpace  A=Ac  B=Bc  C=Cc  D=Dc  InitialCondition=x0c
  Out1 : Outport  VectorParamsAs1DForOutWhenUnconnected=off
  wires:
  In1/1 -> State-Space/1
  State-Space/1 -> Out1/1

== system IEEE34_SPSload/SM_IEEE34/DL_834-860/Load B2/model/PLL/adaptive filter ==
  u : Inport
  freq (Hz) : Inport  Port=2
  Gain : Gain  Gain=2*pi*2*0.707*2
  Gain1 : Gain  Gain=2*pi*2
  Product1 : Product  Inputs=***  RndMeth=Zero
  Product2 : Product  Inputs=**  RndMeth=Zero
  Product3 : Product  Inputs=***  RndMeth=Zero
  Sum1 : Sum  Inputs=+--  InputSameDT=on  SaturateOnIntegerOverflow=on  OutDataTypeStr=Inherit: Same as first input
  integrator1 : Integrator
  integrator2 : Integrator
  y : Outport  VectorParamsAs1DForOutWhenUnconnected=off
  wires:
  Product1/1 -> Sum1/2
  u/1 -> Product3/3
  freq (Hz)/1 -> Gain/1, Gain1/1
  Gain1/1 -> Product1/3, Product1/2, Product3/2, Product3/1
  Product3/1 -> Sum1/1
  integrator1/1 -> Product1/1, y/1
  Gain/1 -> Product2/2
  Product2/1 -> Sum1/3
  Sum1/1 -> integrator2/1
  integrator2/1 -> Product2/1, integrator1/1

== system IEEE34_SPSload/SM_IEEE34/DL_834-860/Load B2/model/PLL/adaptive mean ==
  u : Inport
  freq (Hz) : Inport  Port=2
  Fcn : Fcn  Expr=u(1)+1e-6
  Math Function : Math  Operator=reciprocal  SignedPower=on  SaturateOnIntegerOverflow=on
  Product1 : Product  Inputs=**  RndMeth=Zero
  Sum : Sum  Inputs=+-  InputSameDT=on  SaturateOnIntegerOverflow=on  OutDataTypeStr=Inherit: Same as first input
  Variable Transport Delay : VariableTransportDelay  MaximumDelay=1/40  MaximumPoints=4096
  integrator : Integrator
  y : Outport  VectorParamsAs1DForOutWhenUnconnected=off
  wires:
  Product1/1 -> y/1
  u/1 -> integrator/1
  Sum/1 -> Product1/1
  integrator/1 -> Variable Transport Delay/1, Sum/1
  Variable Transport Delay/1 -> Sum/2
  Math Function/1 -> Variable Transport Delay/2
  freq (Hz)/1 -> Fcn/1
  Fcn/1 -> Math Function/1, Product1/2

== system IEEE34_SPSload/SM_IEEE34/DL_834-860/Load B2/model/Positive Sequence current/TF_P ==
  In1 : Inport
  State-Space : StateSpace  A=Ac  B=Bc  C=Cc  D=Dc  InitialCondition=x0c
  Out1 : Outport  VectorParamsAs1DForOutWhenUnconnected=off
  wires:
  State-Space/1 -> Out1/1
  In1/1 -> State-Space/1

== system IEEE34_SPSload/SM_IEEE34/DL_834-860/Load B2/model/Positive Sequence current/TF_Q ==
  In1 : Inport
  State-Space : StateSpace  A=Ac  B=Bc  C=Cc  D=Dc  InitialCondition=x0c
  Out1 : Outport  VectorParamsAs1DForOutWhenUnconnected=off
  wires:
  In1/1 -> State-Space/1
  State-Space/1 -> Out1/1

== system IEEE34_SPSload/SM_IEEE34/DL_842-1/Load B/model/PLL/adaptive filter ==
  u : Inport
  freq (Hz) : Inport  Port=2
  Gain : Gain  Gain=2*pi*2*0.707*2
  Gain1 : Gain  Gain=2*pi*2
  Product1 : Product  Inputs=***  RndMeth=Zero
  Product2 : Product  Inputs=**  RndMeth=Zero
  Product3 : Product  Inputs=***  RndMeth=Zero
  Sum1 : Sum  Inputs=+--  InputSameDT=on  SaturateOnIntegerOverflow=on  OutDataTypeStr=Inherit: Same as first input
  integrator1 : Integrator
  integrator2 : Integrator
  y : Outport  VectorParamsAs1DForOutWhenUnconnected=off
  wires:
  integrator2/1 -> integrator1/1, Product2/1
  Sum1/1 -> integrator2/1
  Product2/1 -> Sum1/3
  Gain/1 -> Product2/2
  integrator1/1 -> y/1, Product1/1
  Product3/1 -> Sum1/1
  Gain1/1 -> Product3/1, Product3/2, Product1/2, Product1/3
  freq (Hz)/1 -> Gain1/1, Gain/1
  u/1 -> Product3/3
  Product1/1 -> Sum1/2

== system IEEE34_SPSload/SM_IEEE34/DL_842-1/Load B/model/PLL/adaptive mean ==
  u : Inport
  freq (Hz) : Inport  Port=2
  Fcn : Fcn  Expr=u(1)+1e-6
  Math Function : Math  Operator=reciprocal  SignedPower=on  SaturateOnIntegerOverflow=on
  Product1 : Product  Inputs=**  RndMeth=Zero
  Sum : Sum  Inputs=+-  InputSameDT=on  SaturateOnIntegerOverflow=on  OutDataTypeStr=Inherit: Same as first input
  Variable Transport Delay : VariableTransportDelay  MaximumDelay=1/40  MaximumPoints=4096
  integrator : Integrator
  y : Outport  VectorParamsAs1DForOutWhenUnconnected=off
  wires:
  Fcn/1 -> Product1/2, Math Function/1
  freq (Hz)/1 -> Fcn/1
  Math Function/1 -> Variable Transport Delay/2
  Variable Transport Delay/1 -> Sum/2
  integrator/1 -> Sum/1, Variable Transport Delay/1
  Sum/1 -> Product1/1
  u/1 -> integrator/1
  Product1/1 -> y/1

== system IEEE34_SPSload/SM_IEEE34/DL_842-1/Load B/model/Positive Sequence current/TF_P ==
  In1 : Inport
  State-Space : StateSpace  A=Ac  B=Bc  C=Cc  D=Dc  InitialCondition=x0c
  Out1 : Outport  VectorParamsAs1DForOutWhenUnconnected=off
  wires:
  In1/1 -> State-Space/1
  State-Space/1 -> Out1/1

== system IEEE34_SPSload/SM_IEEE34/DL_842-1/Load B/model/Positive Sequence current/TF_Q ==
  In1 : Inport
  State-Space : StateSpace  A=Ac  B=Bc  C=Cc  D=Dc  InitialCondition=x0c
  Out1 : Outport  VectorParamsAs1DForOutWhenUnconnected=off
  wires:
  State-Space/1 -> Out1/1
  In1/1 -> State-Space/1

== system IEEE34_SPSload/SM_IEEE34/DL_842-844/Load B/model/PLL/adaptive filter ==
  u : Inport
  freq (Hz) : Inport  Port=2
  Gain : Gain  Gain=2*pi*2*0.707*2
  Gain1 : Gain  Gain=2*pi*2
  Product1 : Product  Inputs=***  RndMeth=Zero
  Product2 : Product  Inputs=**  RndMeth=Zero
  Product3 : Product  Inputs=***  RndMeth=Zero
  Sum1 : Sum  Inputs=+--  InputSameDT=on  SaturateOnIntegerOverflow=on  OutDataTypeStr=Inherit: Same as first input
  integrator1 : Integrator
  integrator2 : Integrator
  y : Outport  VectorParamsAs1DForOutWhenUnconnected=off
  wires:
  Product1/1 -> Sum1/2
  u/1 -> Product3/3
  freq (Hz)/1 -> Gain/1, Gain1/1
  Gain1/1 -> Product1/3, Product1/2, Product3/2, Product3/1
  Product3/1 -> Sum1/1
  integrator1/1 -> Product1/1, y/1
  Gain/1 -> Product2/2
  Product2/1 -> Sum1/3
  Sum1/1 -> integrator2/1
  integrator2/1 -> Product2/1, integrator1/1

== system IEEE34_SPSload/SM_IEEE34/DL_842-844/Load B/model/PLL/adaptive mean ==
  u : Inport
  freq (Hz) : Inport  Port=2
  Fcn : Fcn  Expr=u(1)+1e-6
  Math Function : Math  Operator=reciprocal  SignedPower=on  SaturateOnIntegerOverflow=on
  Product1 : Product  Inputs=**  RndMeth=Zero
  Sum : Sum  Inputs=+-  InputSameDT=on  SaturateOnIntegerOverflow=on  OutDataTypeStr=Inherit: Same as first input
  Variable Transport Delay : VariableTransportDelay  MaximumDelay=1/40  MaximumPoints=4096
  integrator : Integrator
  y : Outport  VectorParamsAs1DForOutWhenUnconnected=off
  wires:
  Product1/1 -> y/1
  u/1 -> integrator/1
  Sum/1 -> Product1/1
  integrator/1 -> Variable Transport Delay/1, Sum/1
  Variable Transport Delay/1 -> Sum/2
  Math Function/1 -> Variable Transport Delay/2
  freq (Hz)/1 -> Fcn/1
  Fcn/1 -> Math Function/1, Product1/2

== system IEEE34_SPSload/SM_IEEE34/DL_842-844/Load B/model/Positive Sequence current/TF_P ==
  In1 : Inport
  State-Space : StateSpace  A=Ac  B=Bc  C=Cc  D=Dc  InitialCondition=x0c
  Out1 : Outport  VectorParamsAs1DForOutWhenUnconnected=off
  wires:
  State-Space/1 -> Out1/1
  In1/1 -> State-Space/1

== system IEEE34_SPSload/SM_IEEE34/DL_842-844/Load B/model/Positive Sequence current/TF_Q ==
  In1 : Inport
  State-Space : StateSpace  A=Ac  B=Bc  C=Cc  D=Dc  InitialCondition=x0c
  Out1 : Outport  VectorParamsAs1DForOutWhenUnconnected=off
  wires:
  In1/1 -> State-Space/1
  State-Space/1 -> Out1/1

== system IEEE34_SPSload/SM_IEEE34/DL_844-1/Load B/model/PLL/adaptive filter ==
  u : Inport
  freq (Hz) : Inport  Port=2
  Gain : Gain  Gain=2*pi*2*0.707*2
  Gain1 : Gain  Gain=2*pi*2
  Product1 : Product  Inputs=***  RndMeth=Zero
  Product2 : Product  Inputs=**  RndMeth=Zero
  Product3 : Product  Inputs=***  RndMeth=Zero
  Sum1 : Sum  Inputs=+--  InputSameDT=on  SaturateOnIntegerOverflow=on  OutDataTypeStr=Inherit: Same as first input
  integrator1 : Integrator
  integrator2 : Integrator
  y : Outport  VectorParamsAs1DForOutWhenUnconnected=off
  wires:
  integrator2/1 -> integrator1/1, Product2/1
  Sum1/1 -> integrator2/1
  Product2/1 -> Sum1/3
  Gain/1 -> Product2/2
  integrator1/1 -> y/1, Product1/1
  Product3/1 -> Sum1/1
  Gain1/1 -> Product3/1, Product3/2, Product1/2, Product1/3
  freq (Hz)/1 -> Gain1/1, Gain/1
  u/1 -> Product3/3
  Product1/1 -> Sum1/2
